simulink model "aerodynamic_model"  (R2025b)
settings: Solver=FixedStepAuto  StartTime=0  StopTime=100  FixedStep=0.001  RelTol=1e-3  EnableMultiTasking=on
model workspace (MAT data in the model file):
  cycleAvg = 0
  wing_alpha = 0.785398163397
libraries: matrix_library x2, dspstat3 x2, vrlib x2
settings Model: DataDictionary=pid.sldd  EnableAccessToBaseWorkspace=off  ModifiedByFormat=The MathWorks Inc.  ParameterArgumentNames=cycleAvg  Creator=The MathWorks, Inc.  LastModifiedBy=The MathWorks Inc.
settings SolverCC: AlgebraicLoopSolver=TrustRegion  AutoInsertRateTranBlk=on
settings DataIOCC: SaveFormat=StructureWithTime  ReturnWorkspaceOutputs=off
settings OptimizationCC: BlockReduction=off  DefaultParameterBehavior=Inlined  InlineInvariantSignals=on  BufferReuse=off  PassReuseOutputArgsAs=Individual arguments  ExpressionDepthLimit=2147483647.0  ZeroExternalMemoryAtStartup=off  ZeroInternalMemoryAtStartup=off  EfficientFloat2IntCast=on  LifeSpan=1  EfficientTunableParamExpr=on
settings DebuggingCC: AlgebraicLoopMsg=none  FcnCallInpInsideContextMsg=warning  UniqueDataStoreMsg=error  AssertControl=DisableAll  AllowSymbolicDim=off  StateNameClashWarn=warning  StrictBusMsg=ErrorOnBusTreatedAsVector  SFUnexpectedBacktrackingDiag=warning  SFNoUnconditionalDefaultTransitionDiag=warning  SFExecutionAtInitializationDiag=none  UnderSpecifiedDimensionMsg=warning  ArithmeticOperatorsInVariantConditions=warning
settings HardwareCC: ProdBitPerPointer=32.0  ProdBitPerSizeT=32.0  ProdBitPerPtrDiffT=32.0  ProdLargestAtomicFloat=None  ProdIntDivRoundTo=Undefined  ProdEndianess=Unspecified  ProdWordSize=32.0  ProdHWDeviceType=32-bit Generic
settings ModelReferenceCC: EnableRefExpFcnMdlSchedulingChecks=on  PropagateSignalLabelsOutOfModel=off
settings SFSimCC: SimUseLocalCustomCode=off  CustomCodeUndefinedFunction=UseInterfaceOnly
settings RTWCC: SystemTargetFile=ert.tlc  TemplateMakefile=ert_default_tmf  GenerateReport=on  RTWUseLocalCustomCode=off  IncludeHyperlinkInReport=on  GenerateTraceInfo=on  GenerateTraceReport=on  GenerateTraceReportSl=on  GenerateTraceReportSf=on  GenerateTraceReportEml=on  GenerateCodeMetricsReport=on  GPUComputeCapability=3.5  DLArmComputeVersion=19.05  Description=Embedded Coder
settings CodeAppCC: IgnoreCustomStorageClasses=off  IgnoreTestpoints=on  CustomSymbolStrType=$N$R$M  StateflowObjectComments=on  InternalIdentifier=Classic
settings ERTTargetCC: ERTCustomFileTemplate=example_file_process.tlc  ConvertIfToSwitch=off  SuppressUnreachableDefaultCases=off  DynamicArrayContainerType=coder::array  MultiwordLength=2048.0  GenerateSampleERTMain=on  SupportNonFinite=off  ParenthesesLevel=Maximum
settings ConfigComp: CovMetricSettings=dw  CovSaveCumulativeToWorkspaceVar=on  CovSaveSingleToWorkspaceVar=on  CovExternalEMLEnable=off  CovSFcnEnable=off

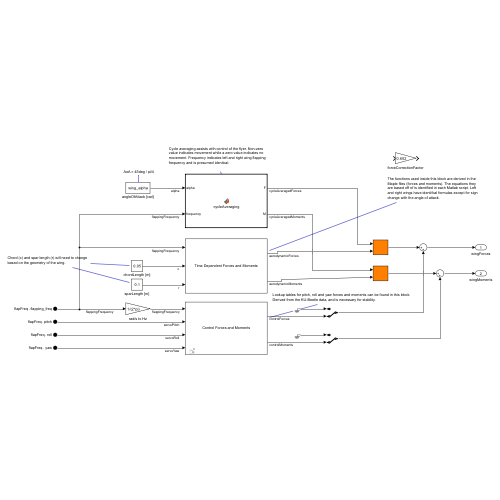
[thumbnail: Simulink's stored preview of the top-level diagram]
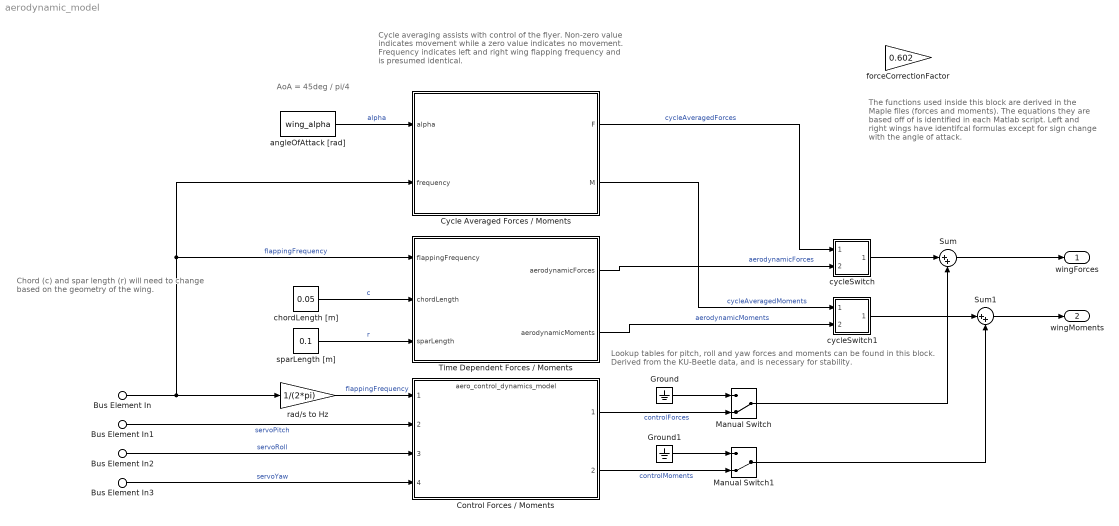
== system aerodynamic_model ==
  note: AoA = 45deg / pi/4
  note: Chord (c) and spar length (r) will need to change
      | based on the geometry of the wing.
  note: Lookup tables for pitch, roll and yaw forces and moments can be found in this block.
      | Derived from the KU-Beetle data, and is necessary for stability.
  note: Cycle averaging assists with control of the flyer. Non-zero
      | value indicates movement while a zero value indicates no
      | movement. Frequency indicates left and right wing flapping
      | frequency and is presumed identical.
  note: The functions used inside this block are derived in the
      | Maple files (forces and moments). The equations they
      | are based off of is identified in each Matlab script. Left
      | and right wings have identifcal formulas except for sign
      | change with the angle of attack.
  Bus Element In : Inport  PortName=flapFreq  Element=flapping_freq
  Bus Element In1 : Inport  PortName=flapFreq  Element=pitch
  Bus Element In2 : Inport  PortName=flapFreq  Element=roll
  Bus Element In3 : Inport  PortName=flapFreq  Element=yaw
  Control Forces / Moments : ModelReference  ModelNameDialog=aero_control_dynamics_model.slx  SimulationMode=Normal  ModelReferenceVersion=10.4
      mask Display: disp('Control Forces and Moments');
  Cycle Averaged Forces / Moments : MATLAB Function  TreatAsAtomicUnit=on
  Ground : Ground
  Ground1 : Ground
  Manual Switch : ManualSwitch  CurrentSetting=0
  Manual Switch1 : ManualSwitch  CurrentSetting=0
  Sum : Sum  Inputs=|++
  Sum1 : Sum  Inputs=|++
  Time Dependent Forces / Moments : Subsystem
      mask Display: disp('Time Dependent Forces and Moments');
  angleOfAttack [rad] : Constant  Value=wing_alpha
  chordLength [m] : Constant  Value=0.05
  cycleSwitch : Subsystem
  cycleSwitch1 : Subsystem
  forceCorrectionFactor : Gain  Gain=0.602
  rad/s to Hz : Gain  Gain=1/(2*pi)
  sparLength [m] : Constant  Value=0.1
  wingForces : Outport  PortDimensions=3
  wingMoments : Outport  Port=2  PortDimensions=3
  wires:
  Bus Element In1/1 -> Control Forces / Moments/2  "servoPitch"
  Bus Element In2/1 -> Control Forces / Moments/3  "servoRoll"
  Bus Element In3/1 -> Control Forces / Moments/4  "servoYaw"
  rad/s to Hz/1 -> Control Forces / Moments/1  "flappingFrequency"
  Sum/1 -> wingForces/1
  Sum1/1 -> wingMoments/1
  Control Forces / Moments/1 -> Manual Switch/2  "controlForces"
  Manual Switch/1 -> Sum/2
  Ground/1 -> Manual Switch/1
  Control Forces / Moments/2 -> Manual Switch1/2  "controlMoments"
  Ground1/1 -> Manual Switch1/1
  Manual Switch1/1 -> Sum1/2
  Bus Element In/1 -> Cycle Averaged Forces / Moments/2(frequency), Time Dependent Forces / Moments/1(flappingFrequency), rad/s to Hz/1  "flappingFrequency"
  angleOfAttack [rad]/1 -> Cycle Averaged Forces / Moments/1(alpha)  "alpha"
  cycleSwitch/1(forces_out) -> Sum/1
  Cycle Averaged Forces / Moments/1(F) -> cycleSwitch/1(cycleAveragedForces_in)  "cycleAveragedForces"
  cycleSwitch1/1(forces_out) -> Sum1/1
  Cycle Averaged Forces / Moments/2(M) -> cycleSwitch1/1(cycleAveragedMoments_in)  "cycleAveragedMoments"
  chordLength [m]/1 -> Time Dependent Forces / Moments/2(chordLength)  "c"
  sparLength [m]/1 -> Time Dependent Forces / Moments/3(sparLength)  "r"
  Time Dependent Forces / Moments/1(aerodynamicForces) -> cycleSwitch/2(aerodynamicForces_in)  "aerodynamicForces"
  Time Dependent Forces / Moments/2(aerodynamicMoments) -> cycleSwitch1/2(aerodynamicMoments_in)  "aerodynamicMoments"

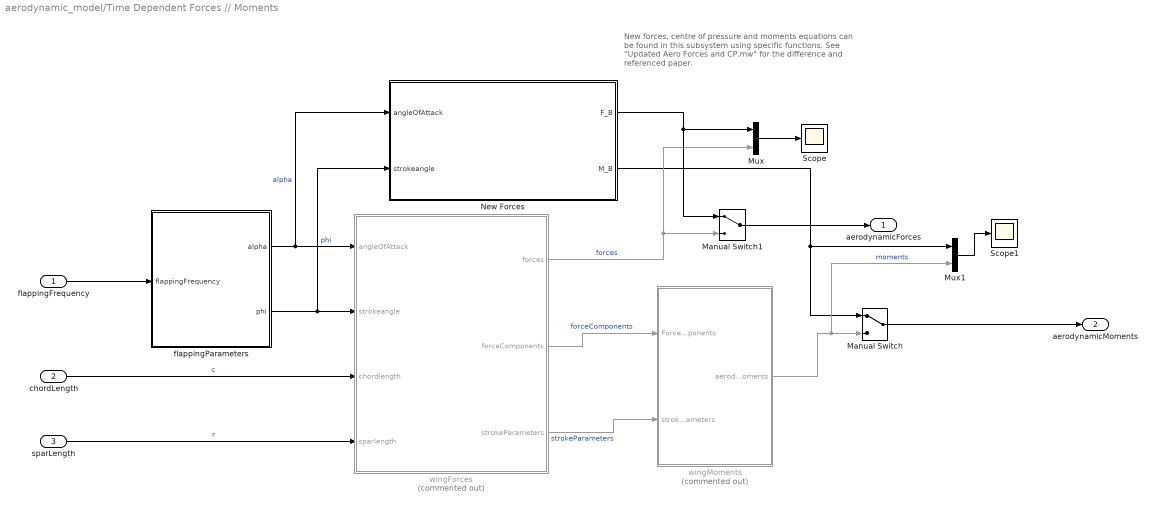
== system aerodynamic_model/Time Dependent Forces // Moments ==
  note: New forces, centre of pressure and moments equations
      | can be found in this subsystem using specific functions.
      | See "Updated Aero Forces and CP.mw" for the difference
      | and referenced paper.
  flappingFrequency : Inport
  chordLength : Inport  Port=2
  sparLength : Inport  Port=3
  Manual Switch : ManualSwitch
  Manual Switch1 : ManualSwitch
  Mux : Mux  Inputs=2
  Mux1 : Mux  Inputs=2
  New Forces : Subsystem
  Scope : Scope
      settings: ActiveDisplayYMinimum=-0.94327179185933741  ActiveDisplayYMaximum=0.98821929568078293  DataLoggingVariableName=ScopeData46
  Scope1 : Scope
      settings: ActiveDisplayYMinimum=-0.082162844612855668  ActiveDisplayYMaximum=0.0814690273769223  DataLoggingVariableName=ScopeData47
  flappingParameters : Subsystem
      mask Display: disp('Flapping Parameters');
  wingForces : Subsystem  Commented=on
      mask Display: disp('Wing Forces');
  wingMoments : Subsystem  Commented=on
      mask Display: disp('Wing Moments');
  aerodynamicForces : Outport
  aerodynamicMoments : Outport  Port=2
  wires:
  flappingParameters/1(alpha) -> New Forces/1(angleOfAttack), wingForces/1(angleOfAttack)  "alpha"
  chordLength/1 -> wingForces/3(chordlength)  "c"
  flappingFrequency/1 -> flappingParameters/1(flappingFrequency)
  flappingParameters/2(phi) -> New Forces/2(strokeangle), wingForces/2(strokeangle)  "phi"
  sparLength/1 -> wingForces/4(sparlength)  "r"
  wingForces/3(strokeParameters) -> wingMoments/2(strokeParameters)  "strokeParameters"
  wingForces/2(forceComponents) -> wingMoments/1(ForceComponents)  "forceComponents"
  New Forces/2(M_B) -> Manual Switch/1, Mux1/1
  Manual Switch/1 -> aerodynamicMoments/1
  wingMoments/1(aerodynamicMoments) -> Mux1/2, Manual Switch/2  "moments"
  Manual Switch1/1 -> aerodynamicForces/1
  wingForces/1(forces) -> Mux/2, Manual Switch1/2  "forces"
  New Forces/1(F_B) -> Mux/1, Manual Switch1/1
  Mux/1 -> Scope/1
  Mux1/1 -> Scope1/1

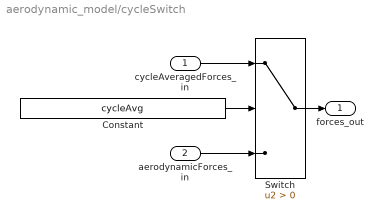
== system aerodynamic_model/cycleSwitch ==
  cycleAveragedForces_in : Inport
  aerodynamicForces_in : Inport  Port=2
  Constant : Constant  Value=cycleAvg
  Switch : Switch  Criteria=u2 > Threshold  SaturateOnIntegerOverflow=off  InputSameDT=off
  forces_out : Outport
  wires:
  Constant/1 -> Switch/2
  aerodynamicForces_in/1 -> Switch/3
  Switch/1 -> forces_out/1
  cycleAveragedForces_in/1 -> Switch/1

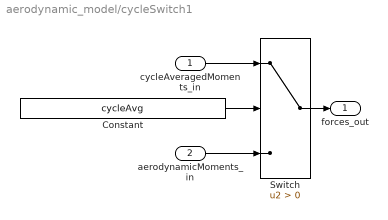
== system aerodynamic_model/cycleSwitch1 ==
  cycleAveragedMoments_in : Inport
  aerodynamicMoments_in : Inport  Port=2
  Constant : Constant  Value=cycleAvg
  Switch : Switch  Criteria=u2 > Threshold  SaturateOnIntegerOverflow=off  InputSameDT=off
  forces_out : Outport
  wires:
  Constant/1 -> Switch/2
  aerodynamicMoments_in/1 -> Switch/3
  Switch/1 -> forces_out/1
  cycleAveragedMoments_in/1 -> Switch/1

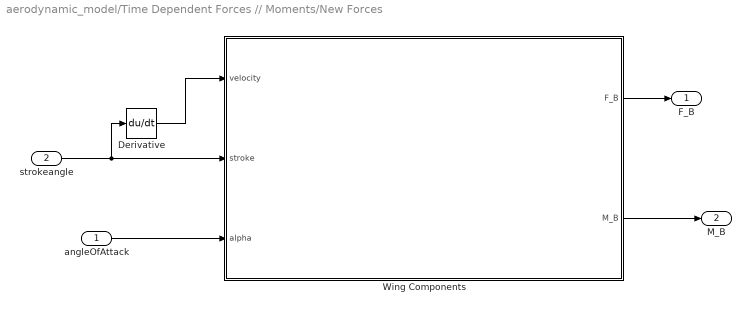
== system aerodynamic_model/Time Dependent Forces // Moments/New Forces ==
  angleOfAttack : Inport
  strokeangle : Inport  Port=2
  Derivative : Derivative
  Wing Components : Subsystem
  F_B : Outport
  M_B : Outport  Port=2
  wires:
  angleOfAttack/1 -> Wing Components/3(alpha)
  Derivative/1 -> Wing Components/1(velocity)
  strokeangle/1 -> Derivative/1, Wing Components/2(stroke)
  Wing Components/1(F_B) -> F_B/1
  Wing Components/2(M_B) -> M_B/1

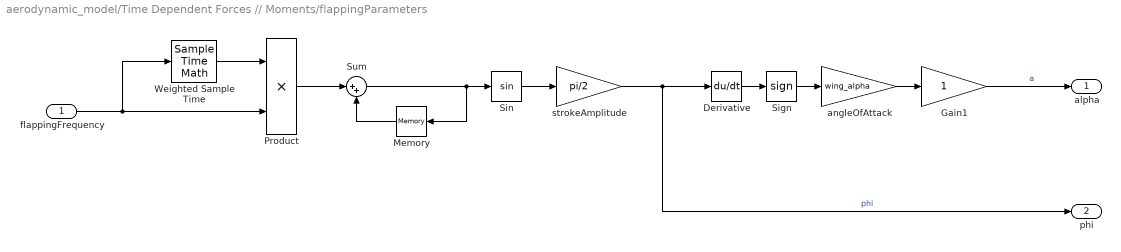
== system aerodynamic_model/Time Dependent Forces // Moments/flappingParameters ==
  flappingFrequency : Inport
  Derivative : Derivative
  Gain1 : Gain
  Memory : Memory
  Product : Product
  Sign : Signum
  Sin : Trigonometry
  Sum : Sum  Inputs=|++
  Weighted Sample Time : SampleTimeMath  TsampMathOp=Ts Only
  angleOfAttack : Gain  Gain=wing_alpha
  strokeAmplitude : Gain  Gain=pi/2
  alpha : Outport
  phi : Outport  Port=2
  wires:
  flappingFrequency/1 -> Product/2, Weighted Sample Time/1
  Product/1 -> Sum/1
  Weighted Sample Time/1 -> Product/1
  Memory/1 -> Sum/2
  Sin/1 -> strokeAmplitude/1
  angleOfAttack/1 -> Gain1/1
  Sum/1 -> Memory/1, Sin/1
  Sign/1 -> angleOfAttack/1
  Derivative/1 -> Sign/1
  strokeAmplitude/1 -> phi/1, Derivative/1  "phi"
  Gain1/1 -> alpha/1  "a"

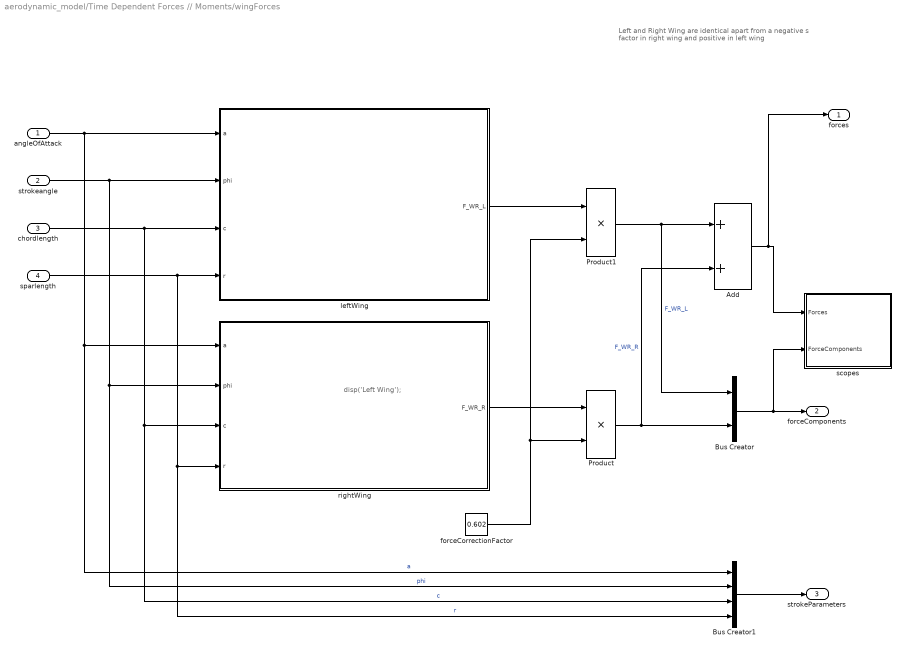
== system aerodynamic_model/Time Dependent Forces // Moments/wingForces ==
  note: Left and Right Wing are identical apart from a negative
      | s factor in right wing and positive in left wing
  note: disp('Left Wing');
  angleOfAttack : Inport
  strokeangle : Inport  Port=2
  chordlength : Inport  Port=3
  sparlength : Inport  Port=4
  Add : Sum
  Bus Creator : BusCreator  Inputs=2
  Bus Creator1 : BusCreator  Inputs=4
  Product : Product
  Product1 : Product
  forceCorrectionFactor : Constant  Value=0.602
  leftWing : Subsystem
      mask Display: disp('Left Wing');
  rightWing : Subsystem
      mask Display: disp('Right Wing');
  scopes : Subsystem
      mask Display: disp('Scopes');
  forces : Outport
  forceComponents : Outport  Port=2
  strokeParameters : Outport  Port=3
  wires:
  strokeangle/1 -> leftWing/2(phi), Bus Creator1/2, rightWing/2(phi)  "phi"
  angleOfAttack/1 -> Bus Creator1/1, rightWing/1(a), leftWing/1(a)  "a"
  Add/1 -> forces/1, scopes/1(Forces)
  chordlength/1 -> leftWing/3(c), Bus Creator1/3, rightWing/3(c)  "c"
  sparlength/1 -> leftWing/4(r), Bus Creator1/4, rightWing/4(r)  "r"
  Bus Creator/1 -> scopes/2(ForceComponents), forceComponents/1
  Product1/1 -> Add/1, Bus Creator/1  "F_WR_L"
  Product/1 -> Bus Creator/2, Add/2  "F_WR_R"
  leftWing/1(F_WR_L) -> Product1/1
  rightWing/1(F_WR_R) -> Product/1
  forceCorrectionFactor/1 -> Product1/2, Product/2
  Bus Creator1/1 -> strokeParameters/1

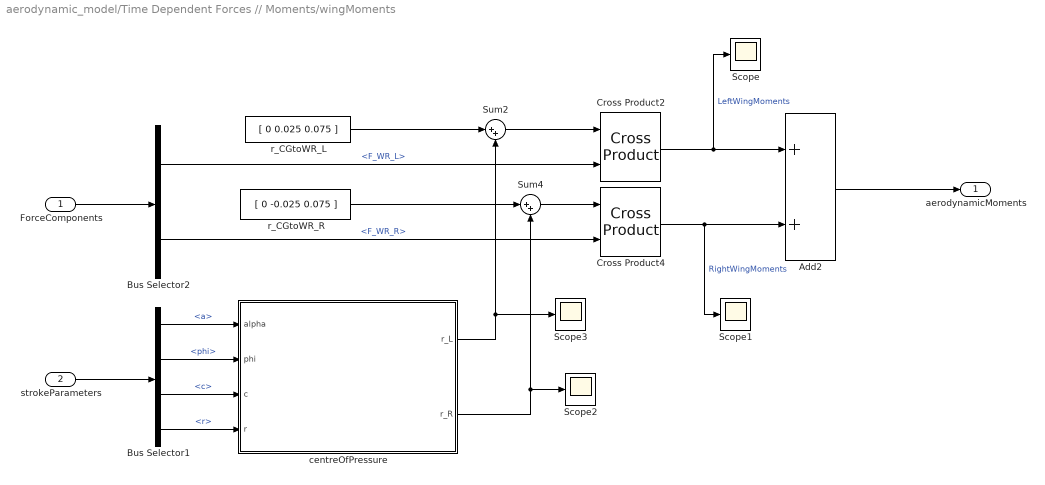
== system aerodynamic_model/Time Dependent Forces // Moments/wingMoments ==
  ForceComponents : Inport
  strokeParameters : Inport  Port=2
  Add2 : Sum
  Bus Selector1 : BusSelector  OutputSignals=a,phi,c,r
  Bus Selector2 : BusSelector  OutputSignals=F_WR_L,F_WR_R
  Cross Product2 : vrlib/Utilities/Cross Product
  Cross Product4 : vrlib/Utilities/Cross Product
  Scope{,1..3} (4 alike) : Scope
      Scope settings: ActiveDisplayYMinimum=-0.041924405683305362  ActiveDisplayYMaximum=0.041936427419196766  DataLoggingVariableName=ScopeData7
      Scope1 settings: ActiveDisplayYMinimum=-0.041924405683305362  ActiveDisplayYMaximum=0.041936427419196766  DataLoggingVariableName=ScopeData8
      Scope2 settings: ActiveDisplayYMinimum=-0.066291260722963027  ActiveDisplayYMaximum=0.06629126072471303  DataLoggingVariableName=ScopeData9
      Scope3 settings: ActiveDisplayYMinimum=-0.066291260649176745  ActiveDisplayYMaximum=0.066291260716514547  DataLoggingVariableName=ScopeData10
  Sum2 : Sum  Inputs=|++
  Sum4 : Sum  Inputs=|++
  centreOfPressure : MATLAB Function  TreatAsAtomicUnit=on
  r_CGtoWR_L : Constant  Value=[ 0 0.025 0.075 ]
  r_CGtoWR_R : Constant  Value=[ 0 -0.025 0.075 ]
  aerodynamicMoments : Outport
  wires:
  strokeParameters/1 -> Bus Selector1/1
  Bus Selector1/1 -> centreOfPressure/1(alpha)  "<a>"
  Bus Selector1/2 -> centreOfPressure/2(phi)  "<phi>"
  Bus Selector1/3 -> centreOfPressure/3(c)  "<c>"
  Bus Selector1/4 -> centreOfPressure/4(r)  "<r>"
  Add2/1 -> aerodynamicMoments/1
  Bus Selector2/1 -> Cross Product2/2  "<F_WR_L>"
  ForceComponents/1 -> Bus Selector2/1
  r_CGtoWR_R/1 -> Sum4/1
  Sum4/1 -> Cross Product4/1
  Cross Product4/1 -> Scope1/1, Add2/2  "RightWingMoments"
  centreOfPressure/1(r_L) -> Sum2/2, Scope3/1
  Bus Selector2/2 -> Cross Product4/2  "<F_WR_R>"
  r_CGtoWR_L/1 -> Sum2/1
  Sum2/1 -> Cross Product2/1
  centreOfPressure/2(r_R) -> Sum4/2, Scope2/1
  Cross Product2/1 -> Scope/1, Add2/1  "LeftWingMoments"

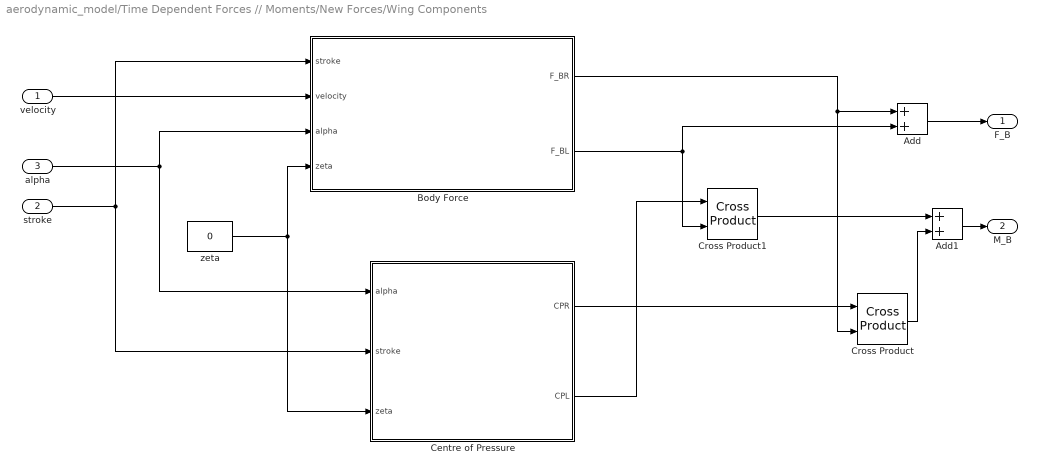
== system aerodynamic_model/Time Dependent Forces // Moments/New Forces/Wing Components ==
  velocity : Inport
  stroke : Inport  Port=2
  alpha : Inport  Port=3
  Add : Sum
  Add1 : Sum
  Body Force : MATLAB Function  TreatAsAtomicUnit=on
  Centre of Pressure : MATLAB Function  TreatAsAtomicUnit=on
  Cross Product : matrix_library/Cross Product
  Cross Product1 : matrix_library/Cross Product
  zeta : Constant  Value=0
  F_B : Outport
  M_B : Outport  Port=2
  wires:
  Centre of Pressure/1(CPR) -> Cross Product/1
  alpha/1 -> Body Force/3(alpha), Centre of Pressure/1(alpha)
  stroke/1 -> Centre of Pressure/2(stroke), Body Force/1(stroke)
  velocity/1 -> Body Force/2(velocity)
  Body Force/1(F_BR) -> Add/1, Cross Product/2
  Centre of Pressure/2(CPL) -> Cross Product1/1
  Body Force/2(F_BL) -> Cross Product1/2, Add/2
  Add/1 -> F_B/1
  Cross Product1/1 -> Add1/1
  Cross Product/1 -> Add1/2
  Add1/1 -> M_B/1
  zeta/1 -> Centre of Pressure/3(zeta), Body Force/4(zeta)

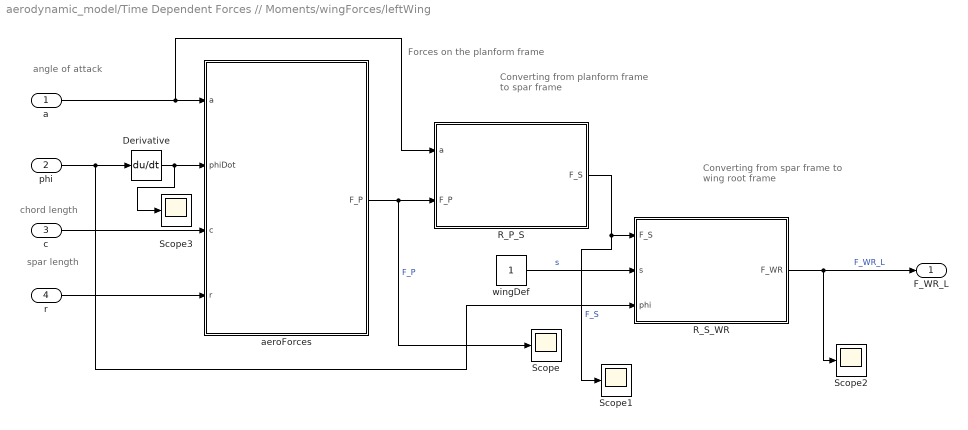
== system aerodynamic_model/Time Dependent Forces // Moments/wingForces/leftWing ==
  note: Converting from spar frame to
      | wing root frame
  note: Converting from planform frame
      | to spar frame
  note: Forces on the planform frame
  note: spar length
  note: chord length
  note: angle of attack
  a : Inport
  phi : Inport  Port=2
  c : Inport  Port=3
  r : Inport  Port=4
  Derivative : Derivative
  R_P_S : MATLAB Function  TreatAsAtomicUnit=on
  R_S_WR : MATLAB Function  TreatAsAtomicUnit=on
  Scope{,1..3} (4 alike) : Scope
      Scope settings: ActiveDisplayYMinimum=-1  ActiveDisplayYMaximum=1  DataLoggingVariableName=ScopeData15
      Scope1 settings: ActiveDisplayYMinimum=-1  ActiveDisplayYMaximum=1  DataLoggingVariableName=ScopeData16
      Scope2 settings: ActiveDisplayYMinimum=-1  ActiveDisplayYMaximum=1  DataLoggingVariableName=ScopeData17
      Scope3 settings: ActiveDisplayYMinimum=-1  ActiveDisplayYMaximum=1  DataLoggingVariableName=ScopeData18
  aeroForces : MATLAB Function  TreatAsAtomicUnit=on
  wingDef : Constant
  F_WR_L : Outport
  wires:
  a/1 -> R_P_S/1(a), aeroForces/1(a)
  c/1 -> aeroForces/3(c)
  aeroForces/1(F_P) -> Scope/1, R_P_S/2(F_P)  "F_P"
  R_P_S/1(F_S) -> Scope1/1, R_S_WR/1(F_S)  "F_S"
  wingDef/1 -> R_S_WR/2(s)  "s"
  phi/1 -> R_S_WR/3(phi), Derivative/1
  r/1 -> aeroForces/4(r)
  Derivative/1 -> Scope3/1, aeroForces/2(phiDot)
  R_S_WR/1(F_WR) -> Scope2/1, F_WR_L/1  "F_WR_L"

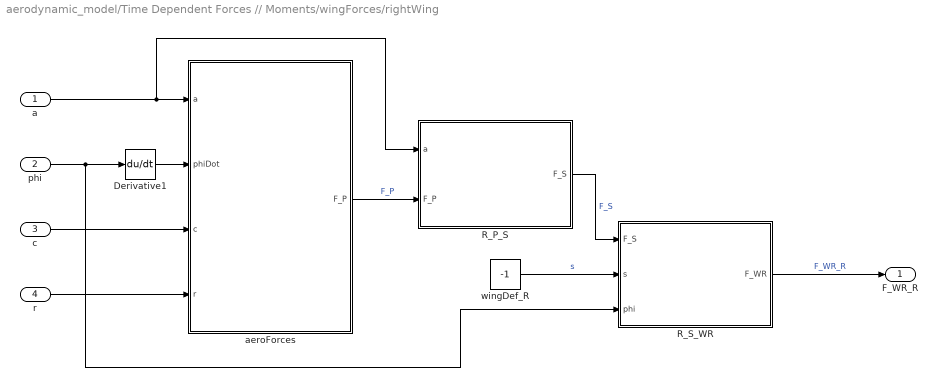
== system aerodynamic_model/Time Dependent Forces // Moments/wingForces/rightWing ==
  a : Inport
  phi : Inport  Port=2
  c : Inport  Port=3
  r : Inport  Port=4
  Derivative1 : Derivative
  R_P_S : MATLAB Function  TreatAsAtomicUnit=on
  R_S_WR : MATLAB Function  TreatAsAtomicUnit=on
  aeroForces : MATLAB Function  TreatAsAtomicUnit=on
  wingDef_R : Constant  Value=-1
  F_WR_R : Outport
  wires:
  aeroForces/1(F_P) -> R_P_S/2(F_P)  "F_P"
  Derivative1/1 -> aeroForces/2(phiDot)
  c/1 -> aeroForces/3(c)
  wingDef_R/1 -> R_S_WR/2(s)  "s"
  R_S_WR/1(F_WR) -> F_WR_R/1  "F_WR_R"
  a/1 -> R_P_S/1(a), aeroForces/1(a)
  R_P_S/1(F_S) -> R_S_WR/1(F_S)  "F_S"
  r/1 -> aeroForces/4(r)
  phi/1 -> R_S_WR/3(phi), Derivative1/1

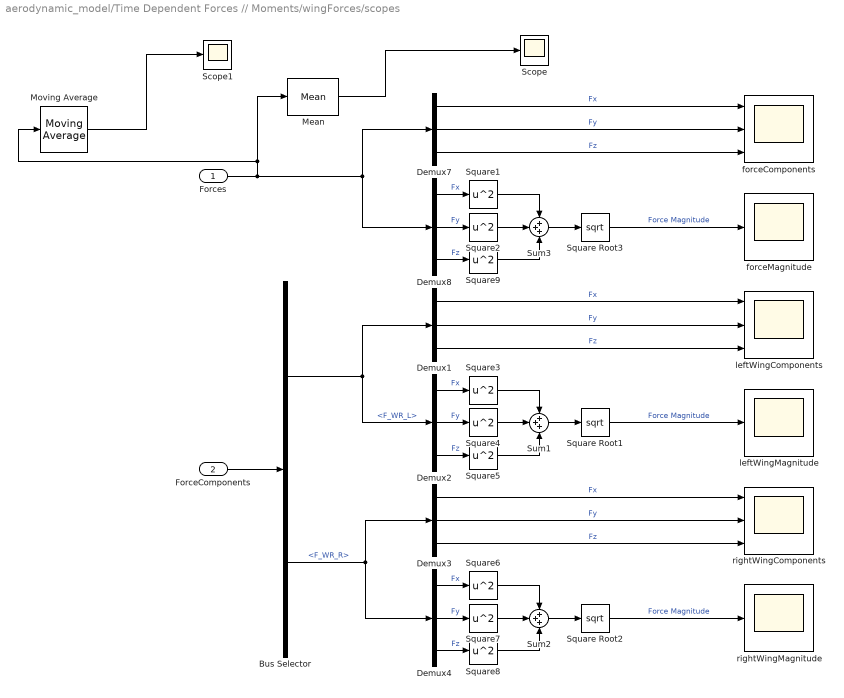
== system aerodynamic_model/Time Dependent Forces // Moments/wingForces/scopes ==
  Forces : Inport
  ForceComponents : Inport  Port=2
  Bus Selector : BusSelector  OutputSignals=F_WR_L,F_WR_R
  Demux{1..4,7..8} (6 alike) : Demux  Outputs=3
  Mean : dspstat3/Mean  run=off  InputProcessing=Columns as channels (frame based)  reset_popup=None  directionMode=Each column  dimension=1  roiEnable=off  roiType=Rectangles  roiPortion=Entire ROI  roiOutput=Individual statistics for each ROI  roiFlag=off  roundingMode=Floor  overflowMode=off  outputDataTypeStr=Inherit: Same as accumulator  outputMin=[]  outputMax=[]  outputLastDataTypeStr=Inherit: Same as accumulator
  Moving Average : dspstat3/Moving Average  Method=Sliding window  ForgettingFactorPort=off  SpecifyWindowLength=on  WindowLength=4  OverlapLength=3  AllowArbitraryInputLength=off  ForgettingFactor=0.9  SimulateUsing=Interpreted execution
  Scope : Scope
      settings: ActiveDisplayYMinimum=-0.065393031769189688  ActiveDisplayYMaximum=0.58853728592270738  DataLoggingVariableName=ScopeData33
  Scope1 : Scope
      settings: ActiveDisplayYMinimum=-0.23807668707484811  ActiveDisplayYMaximum=0.23809087423473962  DataLoggingVariableName=ScopeData34
  Square Root1 : Sqrt
  Square Root2 : Sqrt
  Square Root3 : Sqrt
  Square{1..9} (9 alike) : Math  Operator=square
  Sum1 : Sum  Inputs=+++
  Sum2 : Sum  Inputs=+++
  Sum3 : Sum  Inputs=+++
  forceComponents : Scope  NumInputPorts=3
      settings: ActiveDisplayYMinimum=-1.2924332828752099  ActiveDisplayYMaximum=1.2927916825453105
  forceMagnitude : Scope
      settings: ActiveDisplayYMinimum=-0.15615564765103931  ActiveDisplayYMaximum=1.405400828859354  DataLoggingVariableName=ScopeData2
  leftWingComponents : Scope  NumInputPorts=3
      settings: ActiveDisplayYMinimum=-0.53556579078911293  ActiveDisplayYMaximum=0.53561620829000134  DataLoggingVariableName=ScopeData3
  leftWingMagnitude : Scope
      settings: ActiveDisplayYMinimum=-0.078194507544439171  ActiveDisplayYMaximum=0.70375056789995272  DataLoggingVariableName=ScopeData4
  rightWingComponents : Scope  NumInputPorts=3
      settings: ActiveDisplayYMinimum=-0.53556579078911293  ActiveDisplayYMaximum=0.53561620829000134  DataLoggingVariableName=ScopeData5
  rightWingMagnitude : Scope
      settings: ActiveDisplayYMinimum=-0.326  ActiveDisplayYMaximum=2.93403  DataLoggingVariableName=ScopeData6
  wires:
  Forces/1 -> Mean/1, Moving Average/1, Demux8/1, Demux7/1
  Demux8/3 -> Square9/1  "Fz"
  Square Root3/1 -> forceMagnitude/1  "Force Magnitude"
  Square1/1 -> Sum3/1
  Square2/1 -> Sum3/2
  Demux7/1 -> forceComponents/1  "Fx"
  Demux7/2 -> forceComponents/2  "Fy"
  Demux7/3 -> forceComponents/3  "Fz"
  Demux8/2 -> Square2/1  "Fy"
  Demux8/1 -> Square1/1  "Fx"
  Sum3/1 -> Square Root3/1
  Square9/1 -> Sum3/3
  Square5/1 -> Sum1/3
  Sum1/1 -> Square Root1/1
  Demux2/1 -> Square3/1  "Fx"
  Demux2/2 -> Square4/1  "Fy"
  Demux1/3 -> leftWingComponents/3  "Fz"
  Demux1/2 -> leftWingComponents/2  "Fy"
  Demux1/1 -> leftWingComponents/1  "Fx"
  Square4/1 -> Sum1/2
  Square3/1 -> Sum1/1
  Square Root1/1 -> leftWingMagnitude/1  "Force Magnitude"
  Demux2/3 -> Square5/1  "Fz"
  ForceComponents/1 -> Bus Selector/1
  Bus Selector/1 -> Demux2/1, Demux1/1  "<F_WR_L>"
  Demux4/3 -> Square8/1  "Fz"
  Square Root2/1 -> rightWingMagnitude/1  "Force Magnitude"
  Square6/1 -> Sum2/1
  Square7/1 -> Sum2/2
  Demux3/1 -> rightWingComponents/1  "Fx"
  Demux3/2 -> rightWingComponents/2  "Fy"
  Demux3/3 -> rightWingComponents/3  "Fz"
  Demux4/2 -> Square7/1  "Fy"
  Demux4/1 -> Square6/1  "Fx"
  Sum2/1 -> Square Root2/1
  Square8/1 -> Sum2/3
  Bus Selector/2 -> Demux4/1, Demux3/1  "<F_WR_R>"
  Mean/1 -> Scope/1
  Moving Average/1 -> Scope1/1

== matlab function aerodynamic_model/Time Dependent Forces // Moments/New Forces/Wing Components/Centre of Pressure ==
  data: CPR output; alpha input; stroke input; CPL output; zeta input
function [CPR,CPL]= CPtoB(alpha,stroke,zeta)

% x_cp = centre of pressure on planform (y_cp) [m]
% delx_B = distance from CG to wing root (w/2, delz_B) [m]

%see Maple file for derivation of z_cp/y_cp
z_cp=0.048478;
y_cp=0.079533;

%purely geometric, depending on how the flyer is constructed (approx.), [m]
delx_B=0.00;
delz_B=0.025;
w=0.04;

CPR = [-z_cp*sin(alpha)*sin(zeta)+ cos(zeta)*(-sign(alpha)*z_cp*cos(stroke)*cos(alpha)+y_cp*sin(stroke))+delx_B;
      -(sign(alpha)*z_cp*sin(stroke)*cos(alpha) + y_cp*cos(stroke) + w/2);
      z_cp*sin(alpha)*cos(zeta)+ sin(zeta)*(-sign(alpha)*z_cp*cos(stroke)*cos(alpha)+y_cp*sin(stroke))+delz_B];

CPL = [-z_cp*sin(alpha)*sin(zeta)+ cos(zeta)*(-sign(alpha)*z_cp*cos(stroke)*cos(alpha)+y_cp*sin(stroke))+delx_B;
      -(-sign(alpha)*z_cp*sin(stroke)*cos(alpha) - y_cp*cos(stroke) - w/2);
      z_cp*sin(alpha)*cos(zeta)+ sin(zeta)*(-sign(alpha)*z_cp*cos(stroke)*cos(alpha)+y_cp*sin(stroke))+delz_B];

== matlab function aerodynamic_model/Time Dependent Forces // Moments/wingForces/leftWing/R_S_WR ==
  data: F_S input; s input; phi input; F_WR output
function F_WR = S_to_WR(F_S,s,phi)

arg = s*phi;

% R_S_WR = [  
%              0          0         -1 ;
%             -sin(arg)  cos(arg)    0 ;
%              cos(arg)  sin(arg)    0 ;
%          ];
R_S_WR = [  
           cos(arg)  -sin(arg)    0 ;
           sin(arg)   cos(arg)    0 ;
              0          0        1 ;
         ];

F_WR = R_S_WR * F_S;

end

== matlab function aerodynamic_model/Time Dependent Forces // Moments/wingForces/leftWing/aeroForces ==
  data: a input; F_P output; phiDot input; c input; r input
function F_P = aeroForces(a,phiDot,c,r)

% Declare sizes
F_P = zeros(3,1);
% Define the density of air [kg/m^3]
p = 1.225; 
% Define the value of the F-P angle theta
theta = -a;

% Define the lift and drag coefficients using the absolute value of alpha
% Found in MFWF_Maple_forceCorrection.mw Eq. 9 & 10
cL = 0.225 + 1.58*sin((2.13*abs(a))-(7.2*(pi()/180)));
cD = 1.92 - 1.55*cos((2.04*abs(a))-(9.82*(pi()/180)));

% Calculate the cartesian components of the force vector in the P frame
% Found in MFWF_Maple_forceCorrection.mw Eq. 27, assuming r1 = 0
Fx_P = (-1/6)*cos(theta)*sign(a)*p*(phiDot^2)*cD*c*(r^3) + (1/6)*sin(theta)*p*(phiDot^2)*cL*c*(r^3);
Fy_P = 0;
Fz_P = (1/6)*sin(theta)*sign(a)*p*(phiDot^2)*cD*c*(r^3) + (1/6)*cos(theta)*p*(phiDot^2)*cL*c*(r^3);

% Construct the force vector in the P frame
% Found in MFWF_Maple_forceCorrection.mw Eq. 27
F_P = [ Fx_P ;
        Fy_P ; 
        Fz_P ; ];

end

== matlab function aerodynamic_model/Time Dependent Forces // Moments/wingForces/leftWing/R_P_S ==
  data: a input; F_P input; F_S output
function F_S = P_to_S(a,F_P)
% Found in MFWF_Maple_forceCorrection.mw Eq. 3
R_P_S = [  
           cos(a)   0   sin(a) ;
             0      1     0    ;
          -sin(a)   0   cos(a) ;
        ];

F_S = R_P_S * F_P;

end

== matlab function aerodynamic_model/Time Dependent Forces // Moments/wingForces/rightWing/R_P_S ==
  data: a input; F_P input; F_S output
function F_S = P_to_S(a,F_P)

R_P_S = [  
           cos(a)   0   sin(a) ;
             0      1     0    ;
          -sin(a)   0   cos(a) ;
        ];

F_S = R_P_S * F_P;

end

== matlab function aerodynamic_model/Time Dependent Forces // Moments/wingForces/rightWing/R_S_WR ==
  data: F_S input; s input; phi input; F_WR output
function F_WR = S_to_WR(F_S,s,phi)
% Found in MFWF_Maple_forceCorrection.mw Eq. 1 as transpose
arg = s*phi;

R_S_WR = [  
           cos(arg)  -sin(arg)    0 ;
           sin(arg)   cos(arg)    0 ;
              0          0        1 ;
         ];

F_WR = R_S_WR * F_S;

end

== matlab function aerodynamic_model/Time Dependent Forces // Moments/wingForces/rightWing/aeroForces ==
  data: a input; F_P output; phiDot input; c input; r input
function F_P = aeroForces(a,phiDot,c,r)

% Declare sizes
F_P = zeros(3,1);

% Define the density of air [kg/m^3]
p = 1.225; 

% Define the value of the F-P angle theta
theta = -a;

% Define the lift and drag coefficients using the absolute value of alpha
cL = 0.225 + 1.58*sin((2.13*abs(a))-(7.2*(pi()/180)));
cD = 1.92 - 1.55*cos((2.04*abs(a))-(9.82*(pi()/180)));

% Calculate the cartesian components of the force vector in the P frame
Fx_P = (-1/6)*cos(theta)*sign(a)*p*(phiDot^2)*cD*c*(r^3) + (1/6)*sin(theta)*p*(phiDot^2)*cL*c*(r^3);
Fy_P = 0;
Fz_P = (1/6)*sin(theta)*sign(a)*p*(phiDot^2)*cD*c*(r^3) + (1/6)*cos(theta)*p*(phiDot^2)*cL*c*(r^3);

% Construct the force vector in the P frame
F_P = [ Fx_P ;
        Fy_P ; 
        Fz_P ; ];

end

== matlab function aerodynamic_model/Cycle Averaged Forces // Moments ==
  data: alpha input; F output; frequency input; M output
function [F,M] = cycleAveraging(alpha, frequency)
if frequency > 0
    F = real(cycleAveragedForce(alpha, frequency, frequency));
    M = real(cycleAveragedMoment(alpha, frequency, frequency));
else
    F = [0,0,0];
    M = [0,0,0];

end
% In order to see what is actually going in this function, see the
% associated MATLAB scripts cycleAveragedForce and cycleAverageMoment.
% The explicit equations for x, y and z forces and corresponding moments 
% can be found in the papers from Sigthorsson, Oppenheimer and Doman.
% The cycle-averaged forces can be found in "Cycle-Averaged Forces.mw"
% Maple file, where the x and z have swapped to match our reference frame.

== matlab function aerodynamic_model/Time Dependent Forces // Moments/New Forces/Wing Components/Body Force ==
  data: F_BR output; stroke input; velocity input; alpha input; F_BL output; zeta input
function [F_BR,F_BL]= BodyForces(stroke, velocity, alpha, zeta)

%stroke = cos(omega*t)
%velocity = d(stroke)/dt = -omega*sin(omega*t)
%I_A = second moment of area
%zeta = incline angle
rho = 1.225;
I_A=1.66e-5; %[m^4]

CL = 1.58*sin(2.13*abs(alpha) - 7.2*pi/180) + 0.225;
CD = -1.55*cos(2.04*abs(alpha) - 9.82*pi/180) + 1.92;

L= rho/2*CL*velocity^2*I_A;
D= rho/2*CD*velocity^2*I_A;

F_BR = [-L*sin(zeta)+sign(alpha)*D*cos(stroke)*cos(zeta);
       sign(alpha)*D*sin(stroke);
       L*cos(zeta)+sign(alpha)*D*cos(stroke)*sin(zeta)];

F_BL = [-L*sin(zeta)+sign(alpha)*D*cos(stroke)*cos(zeta);
       -sign(alpha)*D*sin(stroke);
       L*cos(zeta)+sign(alpha)*D*cos(stroke)*sin(zeta)];

== matlab function aerodynamic_model/Time Dependent Forces // Moments/wingMoments/centreOfPressure ==
  data: alpha input; r_L output; phi input; c input; r input; r_R output
function [r_L,r_R] = r_CP(alpha,phi,c,r)

r_L = zeros(3,1);
r_R = zeros(3,1);

% This function generates the distance to the centre of pressure for each
% wing in the wing root frame. This distance is then added to the CG to WR
% distance for each wing to generate the total moment arm. 
%
% The definition of centre of pressure used here is arbitrarily set to be
% the midpoint of the wing. This is an assumption that is expected to be
% improved moving forward, with this script serving as a baseline for
% future work. See the Maple file for more infomation about this
% derivation.

% Found in MFWF_Maple_CentreofPressure.mw Eq. 30
% Left Wing

s = 1;

r_L = [  (1/2)*cos(s*phi)*sin(alpha)*c + (1/2)*sin(s*phi)*s*r ;
        -(1/2)*sin(s*phi)*sin(alpha)*c + (1/2)*cos(s*phi)*s*r ; 
                               -(1/2)*cos(alpha)*c            ;
      ];      

% Right Wing

s = -1;

r_R = [  (1/2)*cos(s*phi)*sin(alpha)*c + (1/2)*sin(s*phi)*s*r ;
        -(1/2)*sin(s*phi)*sin(alpha)*c + (1/2)*cos(s*phi)*s*r ; 
                               -(1/2)*cos(alpha)*c            ;
      ];      
end
